simulink model "enabled_triggered_subsystem_demo"  (R2020b)
settings: Solver=FixedStepAuto  StartTime=0.0  StopTime=100  FixedStep=1  RelTol=1e-3
libraries: simulink x1
settings Model: Creator=Training  LastModifiedBy=Training

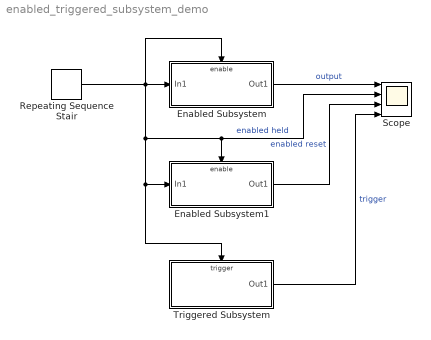
== system enabled_triggered_subsystem_demo ==
  Enabled Subsystem : Subsystem  TreatAsAtomicUnit=on
  Enabled Subsystem1 : Subsystem  TreatAsAtomicUnit=on
  Repeating Sequence Stair : simulink/Sources/Repeating Sequence Stair  OutValues=[0 0 0 1 1 0 1].'  tsamp=-1  OutMin=[]  OutMax=[]  OutDataTypeStr=double  OutputDataTypeScalingMode=double  OutDataType=fixdt(0,8)  ConRadixGroup=Best Precision: Vector-wise  OutScaling=2^-12
  Scope : Scope  NumInputPorts=4
  Triggered Subsystem : Subsystem  TreatAsAtomicUnit=on
  wires:
  Repeating Sequence Stair/1 -> Enabled Subsystem/Enable, Triggered Subsystem/Trigger, Enabled Subsystem1/1(In1), Enabled Subsystem1/Enable, Scope/2, Enabled Subsystem/1(In1)  "enabled held"
  Enabled Subsystem/1(Out1) -> Scope/1  "output"
  Enabled Subsystem1/1(Out1) -> Scope/3  "enabled reset"
  Triggered Subsystem/1(Out1) -> Scope/4  "trigger"

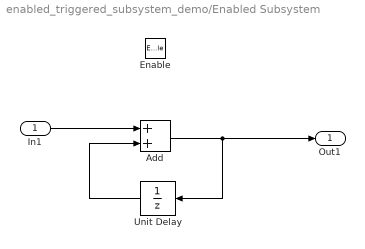
== system enabled_triggered_subsystem_demo/Enabled Subsystem ==
  In1 : Inport
  Enable : EnablePort
  Add : Sum
  Unit Delay : UnitDelay  SampleTime=-1  HasFrameUpgradeWarning=on
  Out1 : Outport
  wires:
  Unit Delay/1 -> Add/2
  Add/1 -> Out1/1, Unit Delay/1
  In1/1 -> Add/1

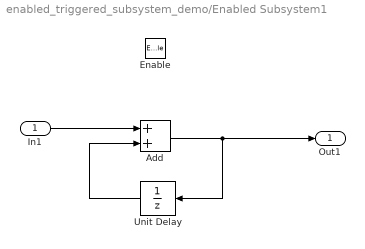
== system enabled_triggered_subsystem_demo/Enabled Subsystem1 ==
  In1 : Inport
  Enable : EnablePort  StatesWhenEnabling=reset
  Add : Sum
  Unit Delay : UnitDelay  SampleTime=-1  HasFrameUpgradeWarning=on
  Out1 : Outport
  wires:
  Unit Delay/1 -> Add/2
  Add/1 -> Out1/1, Unit Delay/1
  In1/1 -> Add/1

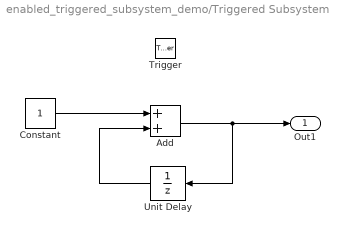
== system enabled_triggered_subsystem_demo/Triggered Subsystem ==
  Trigger : TriggerPort  VariantControl=Variant
  Add : Sum
  Constant : Constant
  Unit Delay : UnitDelay  SampleTime=-1  HasFrameUpgradeWarning=on
  Out1 : Outport
  wires:
  Constant/1 -> Add/1
  Unit Delay/1 -> Add/2
  Add/1 -> Out1/1, Unit Delay/1
